simulink library "ayazLiftingBody_cl"  (R2018b)
settings: Solver=VariableStepAuto  StartTime=0.0  StopTime=10.0  RelTol=1e-3
undefined symbols (not defined in the file or in its folder): ini_euler_ang, ini_O_Vcm_o, ini_OwB, ini_Rcm_o
libraries: thrAttachPtKinematics_ul x3, eulAng2RotMat_ul x1
settings Model: Creator=mcobb  LastModifiedBy=mcobb

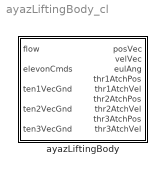
== system ayazLiftingBody_cl ==
  ayazLiftingBody : Subsystem

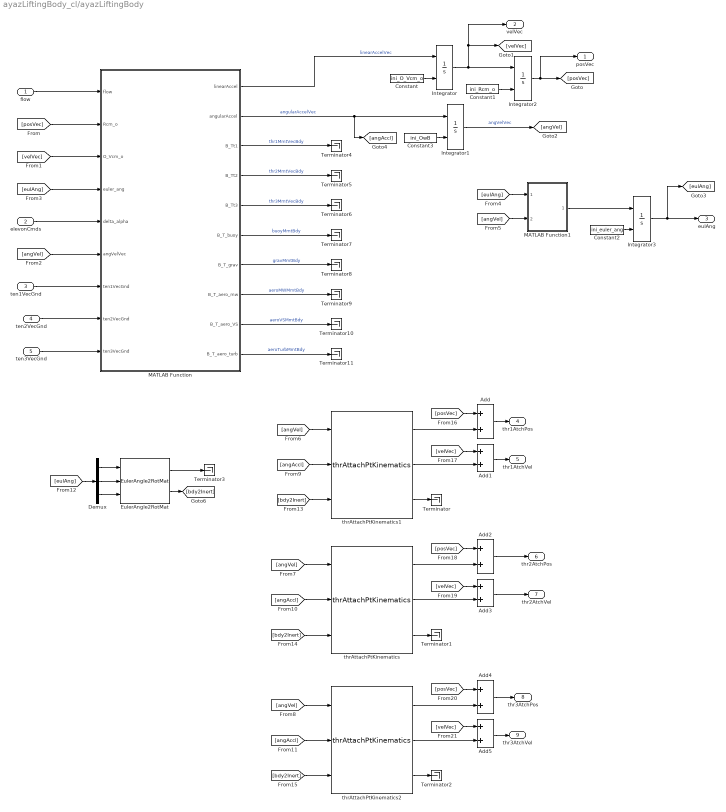
== system ayazLiftingBody_cl/ayazLiftingBody ==
  flow : Inport
  elevonCmds : Inport  Port=2
  ten1VecGnd : Inport  Port=3
  ten2VecGnd : Inport  Port=4
  ten3VecGnd : Inport  Port=5
  Add{,1..5} (6 alike) : Sum
  Constant : Constant  Value=ini_O_Vcm_o
  Constant1 : Constant  Value=ini_Rcm_o
  Constant2 : Constant  Value=ini_euler_ang
  Constant3 : Constant  Value=ini_OwB
  Demux : Demux  Outputs=3
  EulerAngle2RotMat : eulAng2RotMat_ul/EulerAngle2RotMat  SystemSampleTime=-1
  Integrator{,1..3} (4 alike) : Integrator  InitialConditionSource=external
  MATLAB Function : MATLAB Function  TreatAsAtomicUnit=on
  MATLAB Function1 : MATLAB Function  TreatAsAtomicUnit=on
  Terminator{,1..11} (12 alike) : Terminator
  thrAttachPtKinematics : thrAttachPtKinematics_ul/thrAttachPtKinematics  theAtchPosVec=sim_param.tether_imp_nodes.R2n_cm
  thrAttachPtKinematics1 : thrAttachPtKinematics_ul/thrAttachPtKinematics  theAtchPosVec=sim_param.tether_imp_nodes.R1n_cm
  thrAttachPtKinematics2 : thrAttachPtKinematics_ul/thrAttachPtKinematics  theAtchPosVec=sim_param.tether_imp_nodes.R3n_cm
  "posVec " : Outport
  velVec : Outport  Port=2
  eulAng : Outport  Port=3
  thr1AtchPos : Outport  Port=4
  thr1AtchVel : Outport  Port=5
  thr2AtchPos : Outport  Port=6
  thr2AtchVel : Outport  Port=7
  thr3AtchPos : Outport  Port=8
  thr3AtchVel : Outport  Port=9
  wires:
  ten3VecGnd/1 -> MATLAB Function/9(ten3VecGnd)
  ten2VecGnd/1 -> MATLAB Function/8(ten2VecGnd)
  ten1VecGnd/1 -> MATLAB Function/7(ten1VecGnd)
  [eulAng] -> MATLAB Function/4(euler_ang)
  [angVel] -> MATLAB Function/6(angVelVec)
  Integrator3/1 -> eulAng/1, [eulAng]
  [velVec] -> MATLAB Function/3(O_Vcm_o)
  [posVec] -> MATLAB Function/2(Rcm_o)
  Integrator2/1 -> "posVec "/1, [posVec]
  Integrator/1 -> velVec/1, [velVec], Integrator2/1
  Integrator1/1 -> [angVel]  "angVelVec"
  MATLAB Function/2(angularAccel) -> [angAccl], Integrator1/1  "angularAccelVec"
  MATLAB Function/1(linearAccel) -> Integrator/1  "linearAccelVec"
  flow/1 -> MATLAB Function/1(flow)
  elevonCmds/1 -> MATLAB Function/5(delta_alpha)
  Constant/1 -> Integrator/2
  Constant1/1 -> Integrator2/2
  Constant2/1 -> Integrator3/2
  Constant3/1 -> Integrator1/2
  [eulAng] -> MATLAB Function1/1(eulAng)
  [angVel] -> MATLAB Function1/2(angVel)
  MATLAB Function1/1(eulAngDeriv) -> Integrator3/1
  [angVel] -> thrAttachPtKinematics1/1
  [angVel] -> thrAttachPtKinematics/1
  [angVel] -> thrAttachPtKinematics2/1
  [angAccl] -> thrAttachPtKinematics1/2
  [angAccl] -> thrAttachPtKinematics/2
  [angAccl] -> thrAttachPtKinematics2/2
  [eulAng] -> Demux/1
  Demux/2 -> EulerAngle2RotMat/2
  Demux/1 -> EulerAngle2RotMat/1
  Demux/3 -> EulerAngle2RotMat/3
  EulerAngle2RotMat/2 -> [bdy2Inert]
  [bdy2Inert] -> thrAttachPtKinematics1/3
  [bdy2Inert] -> thrAttachPtKinematics/3
  [bdy2Inert] -> thrAttachPtKinematics2/3
  thrAttachPtKinematics1/1 -> Add/2
  thrAttachPtKinematics1/2 -> Add1/2
  thrAttachPtKinematics1/3 -> Terminator/1
  thrAttachPtKinematics/3 -> Terminator1/1
  thrAttachPtKinematics2/3 -> Terminator2/1
  EulerAngle2RotMat/1 -> Terminator3/1
  Add/1 -> thr1AtchPos/1
  [posVec] -> Add/1
  [velVec] -> Add1/1
  Add1/1 -> thr1AtchVel/1
  [velVec] -> Add3/1
  [posVec] -> Add2/1
  thrAttachPtKinematics/2 -> Add3/2
  thrAttachPtKinematics/1 -> Add2/2
  Add2/1 -> thr2AtchPos/1
  Add3/1 -> thr2AtchVel/1
  thrAttachPtKinematics2/1 -> Add4/2
  thrAttachPtKinematics2/2 -> Add5/2
  [posVec] -> Add4/1
  [velVec] -> Add5/1
  Add5/1 -> thr3AtchVel/1
  Add4/1 -> thr3AtchPos/1
  MATLAB Function/3(B_Tt1) -> Terminator4/1  "thr1MmtVecBdy"
  MATLAB Function/4(B_Tt2) -> Terminator5/1  "thr2MmtVecBdy"
  MATLAB Function/5(B_Tt3) -> Terminator6/1  "thr3MmtVecBdy"
  MATLAB Function/7(B_T_grav) -> Terminator8/1  "gravMmtBdy"
  MATLAB Function/8(B_T_aero_mw) -> Terminator9/1  "aeroMWMmtBdy"
  MATLAB Function/9(B_T_aero_VS) -> Terminator10/1  "aeroVSMmtBdy"
  MATLAB Function/10(B_T_aero_turb) -> Terminator11/1  "aeroTurbMmtBdy"
  MATLAB Function/6(B_T_buoy) -> Terminator7/1  "buoyMmtBdy"

== matlab function ayazLiftingBody_cl/ayazLiftingBody/MATLAB Function ==
  data: sim_param parameter; flow input; linearAccel output size=[3 1]; Rcm_o input; O_Vcm_o input; euler_ang input; delta_alpha input; angVelVec input; angularAccel output size=[3 1]; ten1VecGnd input; ten2VecGnd input; ten3VecGnd input; B_Tt1 output; B_Tt2 output; B_Tt3 output; B_T_buoy output; B_T_grav output; B_T_aero_mw output; B_T_aero_VS output; B_T_aero_turb output
function [linearAccel, angularAccel,B_Tt1,B_Tt2,B_Tt3,B_T_buoy,...
    B_T_grav,B_T_aero_mw,B_T_aero_VS,B_T_aero_turb] = ...
    B_F_and_T_aero(sim_param,flow,Rcm_o,O_Vcm_o,euler_ang,delta_alpha,angVelVec,ten1VecGnd,ten2VecGnd,...
    ten3VecGnd)

env_param = sim_param.env_param;
geom_param = sim_param.geom_param;
aero_param = sim_param.aero_param;
turbine_param = sim_param.turbine_param;
tether_param = sim_param.tether_param;
tether_imp_nodes = sim_param.tether_imp_nodes;

m = geom_param.mass;
m_added = geom_param.m_added;
g = env_param.grav;

Rcb_cm = geom_param.center_of_buoy;

R1n_cm = tether_imp_nodes.R1n_cm;
R2n_cm = tether_imp_nodes.R2n_cm;
R3n_cm = tether_imp_nodes.R3n_cm;

[oCb,bCo] = rotation_sequence(euler_ang);

% buoyancy force in the ko direction
fz_buoy = geom_param.F_buoy;

% buoyancy force in the O frame
O_F_buoy = [0;0;fz_buoy];

% gravity force in the ko direction
fz_grav = -m*g;

% gravity force in the O frame
O_F_grav = [0;0;fz_grav];

% calculate aerodynamic forces on the lifting body
aero_F = B_F_and_T_aero(sim_param,flow,Rcm_o,O_Vcm_o,euler_ang,delta_alpha);

B_F_aero_mw = aero_F.B_F_aero_mw;
B_F_aero_VS = aero_F.B_F_aero_VS;
B_F_turb1 = aero_F.B_F_turb1;
B_F_turb2 = aero_F.B_F_turb2;

B_T_aero_mw = aero_F.B_T_aero_mw;
B_T_aero_VS = aero_F.B_T_aero_VS;
B_T_aero_turb = aero_F.B_T_aero_turb;


O_F_aero_mw = oCb*B_F_aero_mw;
O_F_aero_VS = oCb*B_F_aero_VS;
O_F_turb1 = oCb*B_F_turb1;
O_F_turb2 = oCb*B_F_turb2;

% %% forces acting on the center of mass
O_F_ext = O_F_buoy + O_F_grav + O_F_aero_mw + O_F_aero_VS + O_F_turb1 + O_F_turb2 +...
    ten1VecGnd + ten2VecGnd + ten3VecGnd;

mass_matrix = [1/(m+m_added(1)) 0 0;0 1/(m+m_added(2)) 0;0 0 1/(m+m_added(3))];


linearAccel = oCb*(mass_matrix*bCo*O_F_ext);
B_T_buoy = cross(Rcb_cm,(bCo*O_F_buoy));
% torque due to gravity about CM
B_T_grav = [0;0;0];

% torque due to the three tethers in the B frame
B_Tt1 = cross(R1n_cm,(bCo*ten1VecGnd));
B_Tt2 = cross(R2n_cm,(bCo*ten2VecGnd));
B_Tt3 = cross(R3n_cm,(bCo*ten3VecGnd));

B_T_ext = B_T_buoy + B_T_grav + B_T_aero_mw + B_T_aero_VS + B_T_aero_turb + ...
    B_Tt1 + B_Tt2 + B_Tt3;

Tx = B_T_ext(1);
Ty = B_T_ext(2);
Tz = B_T_ext(3);

wx = angVelVec(1);
wy = angVelVec(2);
wz = angVelVec(3);

MI = sim_param.geom_param.MI;
Ixx = MI(1,1);
Iyy = MI(2,2);
Izz = MI(3,3);
Izz_added = sim_param.geom_param.Izz_added;

angularAccel = [...
    (1/Ixx)*(Tx + (Iyy - Izz)*wy*wz);...
    (1/Iyy)*(Ty + (Izz - Ixx)*wx*wz);...
    (1/(Izz+Izz_added))*(Tz + (Ixx - Iyy)*wx*wy)];

end

== matlab function ayazLiftingBody_cl/ayazLiftingBody/MATLAB Function1 ==
  data: eulAng input; eulAngDeriv output; angVel input
function eulAngDeriv = fcn(eulAng,angVel)

wx = angVel(1);
wy = angVel(2);
wz = angVel(3);

ph = eulAng(1);
th = eulAng(2);

eulAngDeriv = zeros(3,1);
eulAngDeriv(1) = wx + sin(ph)*tan(th)*wy + cos(ph)*tan(th)*wz;
eulAngDeriv(2) = cos(ph)*wy - sin(ph)*wz;
eulAngDeriv(3) = sec(th)*sin(ph)*wy + cos(ph)*sec(th)*wz;
